simulink library "tpm"  (R2021b)
settings: Solver=VariableStepAuto  StartTime=0.0  StopTime=10.0  RelTol=1e-3
undefined symbols (not defined in the file or in its folder): ENUM_AN_LF, ENUM_AN_LR, ENUM_AN_RF, ENUM_AN_RR, ENUM_POWERSTA_OFF, ENUM_POWERSTA_OFFA, ENUM_POWERSTA_OFFC, ENUM_POWERSTA_ON, ENUM_POWERSTA_READY, ENUM_POWERSTA_STANDBY, ENUM_PWRSTASW_OFF, ENUM_PWRSTASW_OFFA, ENUM_PWRSTASW_OFFCHVCHRG, ENUM_PWRSTASW_STANDBY, FALSE, KTPM_Delay_raw8, KTPM_WhlRotDir_enum_ovrdflg, KTPM_WhlRotDir_enum_ovrdval, TRUE, ZERO_FLOAT, ZERO_INT
libraries: simulink x58, hcu_lib x25, $bdroot x18
(part 4 of 8)

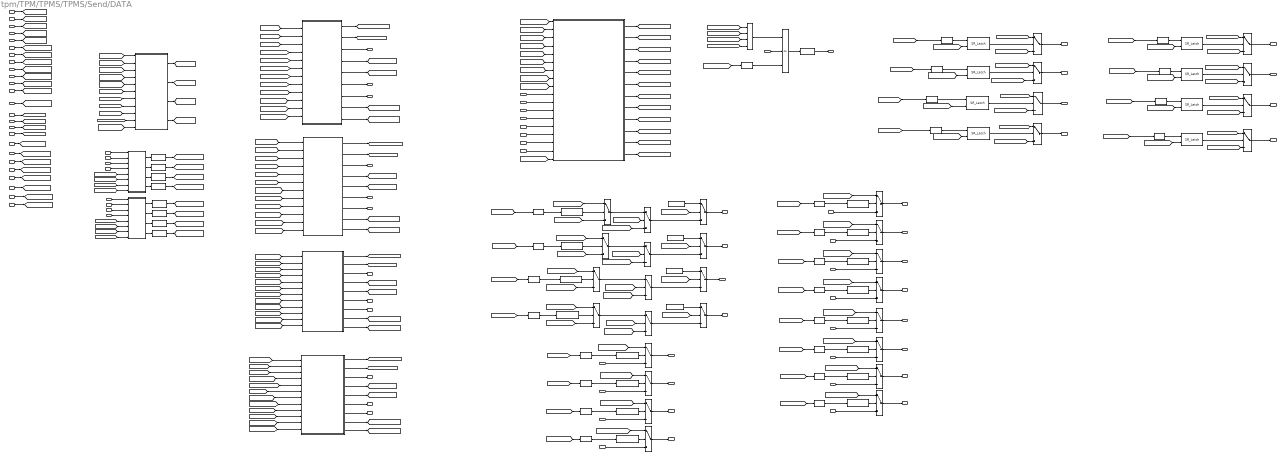
== system tpm/TPM/TPMS/TPMS/Send/DATA ==
  VPMM_PowerSta_enum : Inport
  VTPM_S1ID_raw32 : Inport  Port=2
  VTPM_S2ID_raw32 : Inport  Port=3
  VTPM_S3ID_raw32 : Inport  Port=4
  VTPM_S4ID_raw32 : Inport  Port=5
  VINP_IDin_raw32 : Inport  Port=6
  VINP_DATAin_flg : Inport  Port=7
  VTPM_Done_flg : Inport  Port=8
  VINP_Pin_raw8 : Inport  Port=9
  VINP_Tin_raw8 : Inport  Port=10
  VINP_BatteryLow_flg : Inport  Port=11
  VTPM_S1L_enum : Inport  Port=12
  VTPM_S2L_enum : Inport  Port=13
  VTPM_S3L_enum : Inport  Port=14
  VTPM_S4L_enum : Inport  Port=15
  VINP_FAT_flg : Inport  Port=16
  VINP_VehSpeed_kph : Inport  Port=17
  P1alarm : Inport  Port=18
  P1LowPindi : Inport  Port=19
  P2alarm : Inport  Port=20
  P2LowPindi : Inport  Port=21
  P3alarm : Inport  Port=22
  P3LowPindi : Inport  Port=23
  P4alarm : Inport  Port=24
  P4LowPindi : Inport  Port=25
  VTPM_IDLOCK_flg : Inport  Port=26
  VINP_TPMSResButt_flg : Inport  Port=27
  VINP_FlashLFSensorFail_flg : Inport  Port=28
  VINP_FlashRFSensorFail_flg : Inport  Port=29
  VINP_FlashLRSensorFail_flg : Inport  Port=30
  VINP_FlashRRSensorFail_flg : Inport  Port=31
  VINP_FlashLFWheelPress_raw8 : Inport  Port=32
  VINP_FlashRFWheelPress_raw8 : Inport  Port=33
  VINP_FlashLRFWheelPress_raw8 : Inport  Port=34
  VINP_FlashRRWheelPress_raw8 : Inport  Port=35
  VINP_FlashLFWheelTemp_C : Inport  Port=36
  VINP_FlashRFWheelTemp_C : Inport  Port=37
  VINP_FlashLRWheelTemp_C : Inport  Port=38
  VINP_FlashRRWheelTemp_C : Inport  Port=39
  VINP_FlashLFWheelPSW_raw8 : Inport  Port=40
  VINP_FlashRFWheelPSW_raw8 : Inport  Port=41
  VINP_FlashLRWheelPSW_raw8 : Inport  Port=42
  VINP_FlashRRWheelPSW_raw8 : Inport  Port=43
  VINP_FlashLFPindi_enum : Inport  Port=44
  VINP_FlashRFPindi_enum : Inport  Port=45
  VINP_FlashLRPindi_enum : Inport  Port=46
  VINP_FlashRRPindi_enum : Inport  Port=47
  VINP_FlashLFP20_raw8 : Inport  Port=48
  VINP_FlashRFP20_raw8 : Inport  Port=49
  VINP_FlashLRP20_raw8 : Inport  Port=50
  VINP_FlashRRP20_raw8 : Inport  Port=51
  VTPM_unlearnSfali_flg : Inport  Port=52
  VINP_TPMSCaliButt_flg : Inport  Port=53
  VINP_Prepresstemptrust_flg : Inport  Port=54
  Chart : Stateflow chart  TreatAsAtomicUnit=on
      settings: PortSchema="{\"entries\":[{\"content\":{\"sides\":[{\"content\":{\"connectorIds\":[\"In1\",\"In2\",\"In3\",\"In4\",\"In5\",\"In6\",\"In7\",\"In8\",\"In9\",\"In10\",\"In11\",\"In12\",\"In13\",\"In14\",\"In15\",\"In16\",\"In17\",\"In18\"]},\"type\":\"ConnectorPlacement.EquallySpacedRectSide\",\"uuid\":\"c40bc95c-7acd-49a7-a37f-73ef0237d825\"},{\"content\":{\"connectorIds\":[\"Out1\",\"Out2\",\"Out4\",\"Out3\",\"Out5\",\"Out6\",\"Out7\",\"Out8\",\"Out9\",\"Out10\",\"Out11\",\"Out12\"],\"side\":\"RIGHT\"},\"type\":\"ConnectorPlacement.EquallySpacedRectSide\",\"uuid\":\"6a475380-135f-4803-89fe-753926ba4981\"},{\"content\":{\"connectorIds\":[],\"side\":\"TOP\"},\"type\":\"ConnectorPlacement.EquallySpacedRectSide\",\"uuid\":\"32aff296-3980-42ee-80be-46132fdc59e9\"}]},\"type\":\"ConnectorPlacement.EquallySpacedConnector\",\"uuid\":\"d7f65336-a750-4257-81a4-fde8f4e67659\"}],\"packageUris\":[\"http://schema.mathworks.com/mf0/Connector/R2020b\"],\"version\":\"1.0\"}"
  Constant{1..4} (4 alike) : Constant  Value=TRUE
  Data Type Conversion{4..11,32} (9 alike) : DataTypeConversion  OutDataTypeStr=uint8
  Detect Increase{1..25} (25 alike) : simulink/Logic and Bit Operations/Detect Increase  vinit=0.0  OutDataTypeStr=boolean
  LFSW : Stateflow chart  TreatAsAtomicUnit=on
  LPindSwitch : MATLAB Function  TreatAsAtomicUnit=on
  LRSW : Stateflow chart  TreatAsAtomicUnit=on
      settings: PortSchema="{\"entries\":[{\"content\":{\"sides\":[{\"content\":{\"connectorIds\":[\"In1\",\"In2\",\"In3\",\"In4\",\"In5\",\"In6\",\"In8\",\"In7\",\"In9\",\"In10\",\"In11\",\"In12\"]},\"type\":\"ConnectorPlacement.EquallySpacedRectSide\",\"uuid\":\"46ef0c5c-df75-4382-9dd7-41a48e947ba5\"},{\"content\":{\"connectorIds\":[\"Out1\",\"Out2\",\"Out3\",\"Out4\",\"Out5\",\"Out6\",\"Out7\",\"Out8\",\"Out9\"],\"side\":\"RIGHT\"},\"type\":\"ConnectorPlacement.EquallySpacedRectSide\",\"uuid\":\"b740a0a9-c0c3-4741-b0bb-461f50318db6\"},{\"content\":{\"connectorIds\":[],\"side\":\"TOP\"},\"type\":\"ConnectorPlacement.EquallySpacedRectSide\",\"uuid\":\"ad8490db-8659-4e68-a885-1504b96317d8\"}]},\"type\":\"ConnectorPlacement.EquallySpacedConnector\",\"uuid\":\"0b7e90cb-07df-4d51-93f4-cbf71996ee01\"}],\"packageUris\":[\"http://schema.mathworks.com/mf0/Connector/R2020b\"],\"version\":\"1.0\"}"
  Latch{4..19} (16 alike) : hcu_lib/Basic_Blocks/Latch
  LocationSW : Subsystem
  Logical Operator1 : Logic  Inputs=4  AllPortsSameDT=off  OutDataTypeStr=boolean
  Logical Operator2 : Logic  Operator=OR  Inputs=3  AllPortsSameDT=off  OutDataTypeStr=boolean
  PalarmSwitch : MATLAB Function  TreatAsAtomicUnit=on
  RFSW : Stateflow chart  TreatAsAtomicUnit=on
  RRSW : Stateflow chart  TreatAsAtomicUnit=on
  SR_Latch{,1..7} (8 alike) : hcu_lib/Basic_Blocks/SR_Latch
  Switch{,1..31} (32 alike) : Switch  Criteria=u2 ~= 0
  VTPM_LFWheelPress_raw8 : Outport
  VTPM_LFWheelTemp_C : Outport  Port=2
  VTPM_LFBatWarn_flg : Outport  Port=3
  VTPM_RFWheelPress_raw8 : Outport  Port=4
  VTPM_RFWheelTemp_C : Outport  Port=5
  VTPM_RFBatWarn_flg : Outport  Port=6
  VTPM_LRWheelPress_raw8 : Outport  Port=7
  VTPM_LRWheelTemp_C : Outport  Port=8
  VTPM_LRBatWarn_flg : Outport  Port=9
  VTPM_RRWheelPress_raw8 : Outport  Port=10
  VTPM_RRWheelTemp_C : Outport  Port=11
  VTPM_RRBatWarn_flg : Outport  Port=12
  VTPM_LFWheelDebug_flg : Outport  Port=13
  VTPM_RFWheelDebug_flg : Outport  Port=14
  VTPM_LRWheelDebug_flg : Outport  Port=15
  VTPM_RRWheelDebug_flg : Outport  Port=16
  VTPM_LFSensorMode_flg : Outport  Port=17
  VTPM_RFSensorMode_flg : Outport  Port=18
  VTPM_LRSensorMode_flg : Outport  Port=19
  VTPM_RRSensorMode_flg : Outport  Port=20
  VTPM_LFSensorFail_flg : Outport  Port=21
  VTPM_RFSensorFail_flg : Outport  Port=22
  VTPM_LRSensorFail_flg : Outport  Port=23
  VTPM_RRSensorFail_flg : Outport  Port=24
  VTPM_LFP20_raw8 : Outport  Port=25
  VTPM_RFP20_raw8 : Outport  Port=26
  VTPM_LRP20_raw8 : Outport  Port=27
  VTPM_RRP20_raw8 : Outport  Port=28
  VTPM_LFWheelPSW_raw8 : Outport  Port=29
  VTPM_LFPindi_enum : Outport  Port=30
  VTPM_RFWheelPSW_raw8 : Outport  Port=31
  VTPM_RFPind_enum : Outport  Port=32
  VTPM_LRWheelPSW_raw8 : Outport  Port=33
  VTPM_LRPindi_enum : Outport  Port=34
  VTPM_RRWheelPSW_raw8 : Outport  Port=35
  VTPM_RRPindi_enum : Outport  Port=36
  VTPM_Prepresstempvalid_enum : Outport  Port=37
  wires:
  VINP_Pin_raw8/1 -> [VINP_Pin_raw8]
  VINP_Tin_raw8/1 -> [VINP_Tin_raw8]
  VINP_BatteryLow_flg/1 -> [VINP_BatteryLow_flg]
  LocationSW/1(VTPM_LFSW_flg) -> [VTPM_LFSW_flg]
  LocationSW/2(VTPM_RFSW_flg) -> [VTPM_RFSW_flg]
  LocationSW/3(VTPM_LRSW_flg) -> [VTPM_LRSW_flg]
  LocationSW/4(VTPM_RRSW_flg) -> [VTPM_RRSW_flg]
  VPMM_PowerSta_enum/1 -> [VPMM_PowerSta_enum]
  VINP_DATAin_flg/1 -> [VINP_DATAin_flg]
  VINP_FAT_flg/1 -> [VINP_FAT_flg]
  VINP_VehSpeed_kph/1 -> [VINP_VehSpeed_kph]
  [VINP_FAT_flg] -> LFSW/6(VINP_FAT_flg)
  [VPMM_PowerSta_enum] -> LFSW/5(VPMM_PowerSta_enum)
  [VINP_VehSpeed_kph] -> LFSW/9(VINP_VehSpeed_kph)
  [VTPM_Done_flg] -> LFSW/10(VTPM_Done_flg)
  [VINP_Pin_raw8] -> LFSW/2(VINP_Pin_raw8)
  [VINP_Tin_raw8] -> LFSW/3(VTPM_Tin_c)
  [VTPM_LFSW_flg] -> LFSW/1(VTPM_LFSW_flg)
  [VTPM_LFLowPind_raw] -> LFSW/8(VTPM_S1LowPindi_enum)
  [VINP_BatteryLow_flg] -> LFSW/4(VINP_BatteryLow_flg)
  [VTPM_LFPalarm_raw16] -> LFSW/7(VTPM_LFPalarm_raw16)
  [VTPM_S3L_enum] -> LPindSwitch/7(S3L)
  P4alarm/1 -> PalarmSwitch/4(P4)
  LPindSwitch/2(RFP) -> Data Type Conversion9/1
  [VTPM_S2L_enum] -> PalarmSwitch/6(S2L)
  [VTPM_S4L_enum] -> PalarmSwitch/8(S4L)
  PalarmSwitch/3(LRP) -> Data Type Conversion6/1
  P3LowPindi/1 -> LPindSwitch/3(P3)
  P4LowPindi/1 -> LPindSwitch/4(P4)
  [VTPM_S1L_enum] -> LPindSwitch/5(S1L)
  LPindSwitch/1(LFP) -> Data Type Conversion8/1
  LPindSwitch/4(RRP) -> Data Type Conversion11/1
  [VTPM_S2L_enum] -> LPindSwitch/6(S2L)
  P1LowPindi/1 -> LPindSwitch/1(P1)
  [VTPM_S4L_enum] -> LPindSwitch/8(S4L)
  P1alarm/1 -> PalarmSwitch/1(P1)
  [VTPM_S1L_enum] -> PalarmSwitch/5(S1L)
  PalarmSwitch/1(LFP) -> Data Type Conversion4/1
  [VTPM_S3L_enum] -> PalarmSwitch/7(S3L)
  PalarmSwitch/4(RRP) -> Data Type Conversion7/1
  PalarmSwitch/2(RFP) -> Data Type Conversion5/1
  LPindSwitch/3(LRP) -> Data Type Conversion10/1
  P2alarm/1 -> PalarmSwitch/2(P2)
  P2LowPindi/1 -> LPindSwitch/2(P2)
  P3alarm/1 -> PalarmSwitch/3(P3)
  Data Type Conversion4/1 -> [VTPM_LFPalarm_raw16]
  Data Type Conversion5/1 -> [VTPM_RFPalarm_raw16]
  Data Type Conversion6/1 -> [VTPM_LRPalarm_raw16]
  Data Type Conversion7/1 -> [VTPM_RRPalarm_raw16]
  Data Type Conversion8/1 -> [VTPM_LFLowPind_raw]
  Data Type Conversion9/1 -> [VTPM_RFLowPind_raw]
  Data Type Conversion10/1 -> [VTPM_LRLowPind_raw]
  Data Type Conversion11/1 -> [VTPM_RRLowPind_raw]
  VTPM_S1L_enum/1 -> [VTPM_S1L_enum]
  VTPM_S2L_enum/1 -> [VTPM_S2L_enum]
  VTPM_S3L_enum/1 -> [VTPM_S3L_enum]
  VTPM_S4L_enum/1 -> [VTPM_S4L_enum]
  LFSW/3(VTPM_LFBatWarn_flg) -> VTPM_LFBatWarn_flg/1
  LFSW/6(VTPM_LFWheelDebug_flg) -> VTPM_LFWheelDebug_flg/1
  LFSW/7(VTPM_LFSensorMode_flg) -> VTPM_LFSensorMode_flg/1
  [VINP_DATAin_flg] -> LocationSW/10(VINP_DATAin_flg)
  [VTPM_S1L_enum] -> LocationSW/6(VTPM_S1L_enum)
  [VTPM_S2L_enum] -> LocationSW/7(VTPM_S2L_enum)
  [VTPM_S3L_enum] -> LocationSW/8(VTPM_S3L_enum)
  [VTPM_S4L_enum] -> LocationSW/9(VTPM_S4L_enum)
  VTPM_Done_flg/1 -> [VTPM_Done_flg]
  [VTPM_IDLOCK_flg] -> LocationSW/11(VTPM_IDLOCK_flg)
  VTPM_S1ID_raw32/1 -> [VTPM_S1ID_raw32]
  VTPM_S2ID_raw32/1 -> [VTPM_S2ID_raw32]
  VTPM_S3ID_raw32/1 -> [VTPM_S3ID_raw32]
  VTPM_S4ID_raw32/1 -> [VTPM_S4ID_raw32]
  VINP_IDin_raw32/1 -> [VINP_IDin_raw32]
  [VTPM_S4ID_raw32] -> LocationSW/4(VTPM_S4ID_raw32)
  [VTPM_S3ID_raw32] -> LocationSW/3(VTPM_S3ID_raw32)
  [VINP_IDin_raw32] -> LocationSW/5(VINP_IDin_raw32)
  [VTPM_S2ID_raw32] -> LocationSW/2(VTPM_S2ID_raw32)
  [VTPM_S1ID_raw32] -> LocationSW/1(VTPM_S1ID_raw32)
  [VTPM_S3ID_raw32] -> Chart/4(VTPM_S3ID_raw32)
  [VTPM_S2ID_raw32] -> Chart/3(VTPM_S2ID_raw32)
  [VTPM_S4ID_raw32] -> Chart/5(VTPM_S4ID_raw32)
  [VTPM_S1ID_raw32] -> Chart/2(VTPM_S1ID_raw32)
  [VINP_IDin_raw32] -> Chart/6(VINP_IDin_raw32)
  [VINP_Pin_raw8] -> Chart/8(VINP_Pin_raw8)
  [VINP_DATAin_flg] -> Chart/1(VINP_DATAin_flg)
  VTPM_IDLOCK_flg/1 -> [VTPM_IDLOCK_flg]
  [VTPM_IDLOCK_flg] -> Chart/7(VTPM_IDLOCK_flg)
  [VINP_Tin_raw8] -> Chart/9(VINP_Tin_raw8)
  Chart/1(VTPM_PreS1Pressure_raw) -> [VTPM_PreS1Pressure_raw]
  Chart/2(VTPM_PreS2Pressure_raw) -> [VTPM_PreS2Pressure_raw]
  Chart/5(VTPM_PreS1Temp_raw) -> [VTPM_PreS1Temp_raw]
  Chart/6(VTPM_PreS2Temp_raw) -> [VTPM_PreS2Temp_raw]
  Chart/7(VTPM_PreS3Temp_raw) -> [VTPM_PreS3Temp_raw]
  Chart/8(VTPM_PreS4Temp_raw) -> [VTPM_PreS4Temp_raw]
  Chart/4(VTPM_PreS3Pressure_raw) -> [VTPM_PreS3Pressure_raw]
  Chart/3(VTPM_PreS4Pressure_raw) -> [VTPM_PreS4Pressure_raw]
  LFSW/4(VTPM_LFSensorFail_flg) -> [VTPM_LFSensorFail_flg]
  LFSW/5(VTPM_LFP20_raw8) -> [VTPM_LFP20_raw8]
  LFSW/8(VTPM_LFWheelPSW_raw8) -> [VTPM_LFWheelPSW_raw8]
  LFSW/9(VTPM_LFPindi_enum) -> [VTPM_LFPindi_enum]
  VINP_FlashLFSensorFail_flg/1 -> [VINP_FlashLFSensorFail_flg]
  VINP_FlashRFSensorFail_flg/1 -> [VINP_FlashRFSensorFail_flg]
  VINP_FlashLRSensorFail_flg/1 -> [VINP_FlashLRSensorFail_flg]
  VINP_FlashRRSensorFail_flg/1 -> [VINP_FlashRRSensorFail_flg]
  VINP_FlashLFWheelPress_raw8/1 -> Chart/10(VINP_FlashLFWheelPress_raw8)
  VINP_FlashRFWheelPress_raw8/1 -> Chart/11(VINP_FlashRFWheelPress_raw8)
  VINP_FlashLRFWheelPress_raw8/1 -> Chart/12(VINP_FlashLRWheelPress_raw8)
  VINP_FlashRRWheelPress_raw8/1 -> Chart/13(VINP_FlashRRWheelPress_raw8)
  VINP_FlashLFWheelTemp_C/1 -> Chart/14(VINP_FlashLFWheelTemp_C)
  VINP_FlashRFWheelTemp_C/1 -> Chart/15(VINP_FlashRFWheelTemp_C)
  VINP_FlashLRWheelTemp_C/1 -> Chart/16(VINP_FlashLRWheelTemp_C)
  VINP_FlashRRWheelTemp_C/1 -> Chart/17(VINP_FlashRRWheelTemp_C)
  Switch15/1 -> VTPM_RRPindi_enum/1
  Switch10/1 -> VTPM_LRWheelPSW_raw8/1
  Switch14/1 -> VTPM_LRPindi_enum/1
  Switch11/1 -> VTPM_RRWheelPSW_raw8/1
  Switch4/1 -> VTPM_LFP20_raw8/1
  Switch7/1 -> VTPM_RRP20_raw8/1
  Switch5/1 -> VTPM_RFP20_raw8/1
  Switch8/1 -> VTPM_LFWheelPSW_raw8/1
  Switch13/1 -> VTPM_RFPind_enum/1
  Switch6/1 -> VTPM_LRP20_raw8/1
  Switch9/1 -> VTPM_RFWheelPSW_raw8/1
  Switch12/1 -> VTPM_LFPindi_enum/1
  VINP_FlashRRP20_raw8/1 -> Switch7/3
  VINP_FlashLRPindi_enum/1 -> Switch14/3
  VINP_FlashRRWheelPSW_raw8/1 -> Switch11/3
  VINP_FlashLFWheelPSW_raw8/1 -> Switch8/3
  VINP_FlashRFP20_raw8/1 -> Switch5/3
  VINP_FlashLFP20_raw8/1 -> Switch4/3
  VINP_FlashRRPindi_enum/1 -> Switch15/3
  VINP_FlashRFPindi_enum/1 -> Switch13/3
  VINP_FlashLFPindi_enum/1 -> Switch12/3
  Switch3/1 -> Switch19/1
  Detect Increase4/1 -> Latch4/1
  VINP_FlashRFWheelPSW_raw8/1 -> Switch9/3
  Detect Increase19/1 -> Latch19/1
  [VTPM_LRSW_flg] -> Detect Increase10/1
  [VTPM_RRSW_flg] -> Detect Increase19/1
  Latch13/1 -> Switch9/2
  [VTPM_RRSensorFail_flg] -> Switch19/3
  Latch17/1 -> Switch13/2
  [VTPM_LRPindi_enum] -> Switch14/1
  Latch16/1 -> Switch12/2
  [VTPM_LFP20_raw8] -> Switch4/1
  [VINP_FlashRRSensorFail_flg] -> Switch3/3
  Detect Increase13/1 -> Latch13/1
  [VINP_FlashRRSensorFail_flg] -> Switch19/2
  [VINP_FlashLRSensorFail_flg] -> Switch2/3
  [VTPM_RFPind_enum] -> Switch13/1
  [VTPM_LFSW_flg] -> Detect Increase16/1
  [VTPM_RFSW_flg] -> Detect Increase17/1
  Switch2/1 -> Switch18/1
  [VINP_FlashLRSensorFail_flg] -> Switch18/2
  [VTPM_RFSensorFail_flg] -> Switch1/1
  [VTPM_LRSensorFail_flg] -> Switch18/3
  [VINP_FlashRFSensorFail_flg] -> Switch17/2
  [VINP_FlashRFSensorFail_flg] -> Switch1/3
  [VTPM_RRSensorFail_flg] -> Switch3/1
  Detect Increase8/1 -> Latch8/1
  [VINP_FlashLFSensorFail_flg] -> Switch/3
  Latch9/1 -> Switch5/2
  Detect Increase18/1 -> Latch18/1
  [VTPM_RFSW_flg] -> Detect Increase9/1
  [VTPM_RFSW_flg] -> Detect Increase5/1
  Switch/1 -> Switch16/1
  [VTPM_LFSensorFail_flg] -> Switch16/3
  [VTPM_RFSW_flg] -> Detect Increase13/1
  [VTPM_RRWheelPSW_raw8] -> Switch11/1
  Latch18/1 -> Switch14/2
  Detect Increase14/1 -> Latch14/1
  [VTPM_LRSW_flg] -> Detect Increase18/1
  Detect Increase15/1 -> Latch15/1
  [VTPM_RRSW_flg] -> Detect Increase15/1
  VINP_FlashLRP20_raw8/1 -> Switch6/3
  [VTPM_RFP20_raw8] -> Switch5/1
  [VTPM_RRSW_flg] -> Detect Increase11/1
  Detect Increase17/1 -> Latch17/1
  Detect Increase16/1 -> Latch16/1
  Latch19/1 -> Switch15/2
  Detect Increase10/1 -> Latch10/1
  Latch12/1 -> Switch8/2
  Latch11/1 -> Switch7/2
  Detect Increase9/1 -> Latch9/1
  Latch7/1 -> Switch3/2
  [VTPM_LRSW_flg] -> Detect Increase6/1
  [VTPM_RRP20_raw8] -> Switch7/1
  [VTPM_LFSW_flg] -> Detect Increase8/1
  [VINP_FlashLFSensorFail_flg] -> Switch16/2
  [VTPM_RFWheelPSW_raw8] -> Switch9/1
  Detect Increase11/1 -> Latch11/1
  Detect Increase5/1 -> Latch5/1
  [VTPM_RFSensorFail_flg] -> Switch17/3
  Latch15/1 -> Switch11/2
  Latch6/1 -> Switch2/2
  Latch4/1 -> Switch/2
  Latch14/1 -> Switch10/2
  [VTPM_LRP20_raw8] -> Switch6/1
  Detect Increase6/1 -> Latch6/1
  Switch1/1 -> Switch17/1
  [VTPM_LFPindi_enum] -> Switch12/1
  [VTPM_LRSW_flg] -> Detect Increase14/1
  Latch10/1 -> Switch6/2
  [VTPM_RRPindi_enum] -> Switch15/1
  VINP_FlashLRWheelPSW_raw8/1 -> Switch10/3
  Latch8/1 -> Switch4/2
  [VTPM_LFWheelPSW_raw8] -> Switch8/1
  [VTPM_LFSW_flg] -> Detect Increase4/1
  [VTPM_LFSensorFail_flg] -> Switch/1
  Detect Increase12/1 -> Latch12/1
  [VTPM_LRSensorFail_flg] -> Switch2/1
  [VTPM_LFSW_flg] -> Detect Increase12/1
  Detect Increase7/1 -> Latch7/1
  Latch5/1 -> Switch1/2
  [VTPM_RRSW_flg] -> Detect Increase7/1
  [VTPM_LRWheelPSW_raw8] -> Switch10/1
  VTPM_unlearnSfali_flg/1 -> [VTPM_unlearnSfali_flg]
  Switch16/1 -> Switch20/3
  Switch17/1 -> Switch21/3
  Switch18/1 -> Switch22/3
  Switch19/1 -> Switch23/3
  [VTPM_unlearnSfali_flg] -> Switch20/2
  [VTPM_unlearnSfali_flg] -> Switch21/2
  [VTPM_unlearnSfali_flg] -> Switch22/2
  [VTPM_unlearnSfali_flg] -> Switch23/2
  Constant4/1 -> Switch23/1
  Constant1/1 -> Switch22/1
  Constant2/1 -> Switch21/1
  Constant3/1 -> Switch20/1
  Switch20/1 -> VTPM_LFSensorFail_flg/1
  Switch21/1 -> VTPM_RFSensorFail_flg/1
  Switch22/1 -> VTPM_LRSensorFail_flg/1
  Switch23/1 -> VTPM_RRSensorFail_flg/1
  Data Type Conversion32/1 -> VTPM_Prepresstempvalid_enum/1
  VINP_TPMSCaliButt_flg/1 -> [VINP_TPMSCaliButt_flg]
  VINP_TPMSResButt_flg/1 -> [VINP_TPMSResButt_flg]
  [VINP_TPMSCaliButt_flg] -> LFSW/11(VINP_TPMSCaliButt_flg)
  [VINP_TPMSResButt_flg] -> LFSW/12(VINP_TPMSResButt_flg)
  [VTPM_RFPalarm_raw16] -> RFSW/7(VTPM_P2alarm_raw16)
  [VTPM_RFLowPind_raw] -> RFSW/8(VTPM_S2LowPindi_enum)
  [VINP_VehSpeed_kph] -> RFSW/9(VINP_VehSpeed_kph)
  [VTPM_Done_flg] -> RFSW/10(VTPM_Done_flg)
  [VTPM_RFSW_flg] -> RFSW/1(VTPM_RFSW_flg)
  [VINP_Pin_raw8] -> RFSW/2(VINP_Pin_raw8)
  [VINP_Tin_raw8] -> RFSW/3(VTPM_Tin_c)
  [VINP_BatteryLow_flg] -> RFSW/4(VINP_BatteryLow_flg)
  [VPMM_PowerSta_enum] -> RFSW/5(VPMM_PowerSta_enum)
  [VINP_FAT_flg] -> RFSW/6(VINP_FAT_flg)
  [VTPM_LRSW_flg] -> LRSW/1(VTPM_LRSW_flg)
  [VINP_Pin_raw8] -> LRSW/2(VINP_Pin_raw8)
  [VINP_Tin_raw8] -> LRSW/3(VTPM_Tin_c)
  [VINP_BatteryLow_flg] -> LRSW/4(VINP_BatteryLow_flg)
  [VPMM_PowerSta_enum] -> LRSW/5(VPMM_PowerSta_enum)
  [VINP_FAT_flg] -> LRSW/6(VINP_FAT_flg)
  [VINP_VehSpeed_kph] -> LRSW/9(VINP_VehSpeed_kph)
  [VTPM_Done_flg] -> LRSW/10(VTPM_Done_flg)
  [VTPM_LRPalarm_raw16] -> LRSW/8(VTPM_P3alarm_raw16)
  [VTPM_LRLowPind_raw] -> LRSW/7(VTPM_S3LowPindi_enum)
  [VPMM_PowerSta_enum] -> RRSW/5(VPMM_PowerSta_enum)
  [VTPM_RRLowPind_raw] -> RRSW/8(VTPM_S4LowPindi_enum)
  [VTPM_Done_flg] -> RRSW/10(VTPM_Done_flg)
  [VINP_BatteryLow_flg] -> RRSW/4(VINP_BatteryLow_flg)
  [VINP_VehSpeed_kph] -> RRSW/9(VINP_VehSpeed_kph)
  [VTPM_RRPalarm_raw16] -> RRSW/7(VTPM_P4alarm_raw16)
  [VTPM_RRSW_flg] -> RRSW/1(VTPM_RRSW_flg)
  [VINP_Pin_raw8] -> RRSW/2(VINP_Pin_raw8)
  [VINP_Tin_raw8] -> RRSW/3(VTPM_Tin_c)
  [VINP_FAT_flg] -> RRSW/6(VINP_FAT_flg)
  RFSW/9(VTPM_RFPind_enum) -> [VTPM_RFPind_enum]
  RFSW/3(VTPM_RFBatWarn_flg) -> VTPM_RFBatWarn_flg/1
  RFSW/4(VTPM_RFSensorFail_flg) -> [VTPM_RFSensorFail_flg]
  RFSW/5(VTPM_RFP20_raw8) -> [VTPM_RFP20_raw8]
  RFSW/6(VTPM_RFWheelDebug_flg) -> VTPM_RFWheelDebug_flg/1
  RFSW/7(VTPM_RFSensorMode_flg) -> VTPM_RFSensorMode_flg/1
  RFSW/8(VTPM_RFWheelPSW_raw8) -> [VTPM_RFWheelPSW_raw8]
  LRSW/3(VTPM_LRBatWarn_flg) -> VTPM_LRBatWarn_flg/1
  LRSW/4(VTPM_LRSensorFail_flg) -> [VTPM_LRSensorFail_flg]
  LRSW/5(VTPM_LRP20_raw8) -> [VTPM_LRP20_raw8]
  LRSW/6(VTPM_LRWheelDebug_flg) -> VTPM_LRWheelDebug_flg/1
  LRSW/7(VTPM_LRSensorMode_flg) -> VTPM_LRSensorMode_flg/1
  LRSW/8(VTPM_LRWheelPSW_raw8) -> [VTPM_LRWheelPSW_raw8]
  LRSW/9(VTPM_LRPindi_enum) -> [VTPM_LRPindi_enum]
  RRSW/3(VTPM_RRBatWarn_flg) -> VTPM_RRBatWarn_flg/1
  RRSW/4(VTPM_RRSensorFail_flg) -> [VTPM_RRSensorFail_flg]
  RRSW/5(VTPM_RRP20_raw8) -> [VTPM_RRP20_raw8]
  RRSW/6(VTPM_RRWheelDebug_flg) -> VTPM_RRWheelDebug_flg/1
  RRSW/7(VTPM_RRSensorMode_flg) -> VTPM_RRSensorMode_flg/1
  RRSW/8(VTPM_RRWheelPSW_raw8) -> [VTPM_RRWheelPSW_raw8]
  RRSW/9(VTPM_RRPindi_enum) -> [VTPM_RRPindi_enum]
  [VINP_TPMSCaliButt_flg] -> RFSW/11(VINP_TPMSCaliButt_flg)
  [VINP_TPMSResButt_flg] -> RFSW/12(VINP_TPMSResButt_flg)
  [VINP_TPMSCaliButt_flg] -> LRSW/11(VINP_TPMSCaliButt_flg)
  [VINP_TPMSResButt_flg] -> LRSW/12(VINP_TPMSResButt_flg)
  [VINP_TPMSCaliButt_flg] -> RRSW/11(VINP_TPMSCaliButt_flg)
  [VINP_TPMSResButt_flg] -> RRSW/12(VINP_TPMSResButt_flg)
  [VINP_TPMSResButt_flg] -> Chart/18(VINP_TPMSResButt_flg)
  LFSW/1(VTPM_LFWheelPress_raw8) -> [VTPM_LFWheelPress_raw8]
  LFSW/2(VTPM_LFWheelTemp_C) -> [VTPM_LFWheelTemp_C]
  RFSW/2(VTPM_RFWheelTemp_C) -> [VTPM_RFWheelTemp_C]
  RFSW/1(VTPM_RFWheelPress_raw8) -> [VTPM_RFWheelPress_raw8]
  LRSW/1(VTPM_LRWheelPress_raw8) -> [VTPM_LRWheelPress_raw8]
  LRSW/2(VTPM_LRWheelTemp_C) -> [VTPM_LRWheelTemp_C]
  RRSW/1(VTPM_RRWheelPress_raw8) -> [VTPM_RRWheelPress_raw8]
  RRSW/2(VTPM_RRWheelTemp_C) -> [VTPM_RRWheelTemp_C]
  [VTPM_LFSW_flg] -> Detect Increase21/1
  Detect Increase22/1 -> SR_Latch3/1
  [VTPM_RFSW_flg] -> Detect Increase22/1
  SR_Latch2/1 -> Switch28/2
  [VTPM_PreS1Temp_raw] -> Switch28/3
  [VTPM_PreS1Pressure_raw] -> Switch24/3
  SR_Latch1/1 -> Switch25/2
  Detect Increase21/1 -> SR_Latch2/1
  [VTPM_RFSW_flg] -> Detect Increase2/1
  [VTPM_LFSW_flg] -> Detect Increase1/1
  [VTPM_RFWheelTemp_C] -> Switch29/1
  [VTPM_PreS2Temp_raw] -> Switch29/3
  Detect Increase2/1 -> SR_Latch1/1
  [VTPM_LFWheelPress_raw8] -> Switch24/1
  [VTPM_LFWheelTemp_C] -> Switch28/1
  [VTPM_RFWheelPress_raw8] -> Switch25/1
  [VTPM_PreS2Pressure_raw] -> Switch25/3
  [VTPM_LRWheelPress_raw8] -> Switch26/1
  [VTPM_LRSW_flg] -> Detect Increase3/1
  [VTPM_RRWheelTemp_C] -> Switch31/1
  [VTPM_LRSW_flg] -> Detect Increase23/1
  [VTPM_PreS4Temp_raw] -> Switch31/3
  [VTPM_RRSW_flg] -> Detect Increase24/1
  SR_Latch6/1 -> Switch30/2
  [VTPM_RRWheelPress_raw8] -> Switch27/1
  [VTPM_LRWheelTemp_C] -> Switch30/1
  [VTPM_PreS3Temp_raw] -> Switch30/3
  [VTPM_PreS3Pressure_raw] -> Switch26/3
  [VTPM_PreS4Pressure_raw] -> Switch27/3
  [VTPM_RRSW_flg] -> Detect Increase20/1
  Switch24/1 -> VTPM_LFWheelPress_raw8/1
  Switch28/1 -> VTPM_LFWheelTemp_C/1
  Switch25/1 -> VTPM_RFWheelPress_raw8/1
  Switch29/1 -> VTPM_RFWheelTemp_C/1
  Switch26/1 -> VTPM_LRWheelPress_raw8/1
  Switch30/1 -> VTPM_LRWheelTemp_C/1
  Switch27/1 -> VTPM_RRWheelPress_raw8/1
  Switch31/1 -> VTPM_RRWheelTemp_C/1
  Chart/12(VTPM_PreS4readdone_flg) -> [VTPM_PreS4readdone_flg]
  Chart/11(VTPM_PreS3readdone_flg) -> [VTPM_PreS3readdone_flg]
  Chart/10(VTPM_PreS2readdone_flg) -> [VTPM_PreS2readdone_flg]
  Chart/9(VTPM_PreS1readdone_flg) -> [VTPM_PreS1readdone_flg]
  [VTPM_PreS1readdone_flg] -> Logical Operator1/1
  [VTPM_PreS3readdone_flg] -> Logical Operator1/3
  [VTPM_PreS2readdone_flg] -> Logical Operator1/2
  [VTPM_PreS4readdone_flg] -> Logical Operator1/4
  Logical Operator1/1 -> Logical Operator2/1
  Logical Operator2/1 -> Data Type Conversion32/1
  VINP_Prepresstemptrust_flg/1 -> Logical Operator2/2
  [VINP_TPMSResButt_flg] -> SR_Latch/2
  Detect Increase1/1 -> SR_Latch/1
  SR_Latch/1 -> Switch24/2
  [VINP_TPMSResButt_flg] -> SR_Latch1/2
  [VINP_TPMSResButt_flg] -> SR_Latch2/2
  [VINP_TPMSResButt_flg] -> SR_Latch3/2
  SR_Latch3/1 -> Switch29/2
  [VINP_TPMSResButt_flg] -> SR_Latch4/2
  Detect Increase3/1 -> SR_Latch4/1
  SR_Latch4/1 -> Switch26/2
  [VINP_TPMSResButt_flg] -> SR_Latch5/2
  Detect Increase20/1 -> SR_Latch5/1
  SR_Latch5/1 -> Switch27/2
  [VINP_TPMSResButt_flg] -> SR_Latch6/2
  Detect Increase23/1 -> SR_Latch6/1
  [VINP_TPMSResButt_flg] -> SR_Latch7/2
  Detect Increase24/1 -> SR_Latch7/1
  SR_Latch7/1 -> Switch31/2
  [VINP_TPMSResButt_flg] -> Detect Increase25/1
  Detect Increase25/1 -> Logical Operator2/3

== system tpm/TPM/TPMS/TPMS/Send/ResetAllow&CalibrateAllow ==
  VTQD_GearActualPosn_enum : Inport
  VINP_VehSpeed_kph : Inport  Port=2
  VINP_TPMSResButt_flg : Inport  Port=3
  VINP_TPMSCaliButt_flg : Inport  Port=4
  VTPM_Done_flg : Inport  Port=5
  Chart : Stateflow chart  TreatAsAtomicUnit=on
      settings: PortSchema="{\"entries\":[{\"content\":{\"sides\":[{\"content\":{\"connectorIds\":[\"In1\",\"In2\",\"In3\",\"In4\",\"In5\"]},\"type\":\"ConnectorPlacement.EquallySpacedRectSide\",\"uuid\":\"5043c8d7-7d74-4216-81db-b94b6209e2f2\"},{\"content\":{\"connectorIds\":[\"Out2\",\"Out1\"],\"side\":\"RIGHT\"},\"type\":\"ConnectorPlacement.EquallySpacedRectSide\",\"uuid\":\"32f8b1e1-37fd-4ec2-8559-79f51e6b5aad\"},{\"content\":{\"connectorIds\":[],\"side\":\"TOP\"},\"type\":\"ConnectorPlacement.EquallySpacedRectSide\",\"uuid\":\"4b4c5b66-4800-4ce6-9315-053bf75e645c\"}]},\"type\":\"ConnectorPlacement.EquallySpacedConnector\",\"uuid\":\"baa92019-e8c5-41db-ba73-e08b6ede8e32\"}],\"packageUris\":[\"http://schema.mathworks.com/mf0/Connector/R2020b\"],\"version\":\"1.0\"}"
  VTPM_TPMSResButtAllow_flg : Outport
  VTPM_TPMSCaliButtAllow_flg : Outport  Port=2
  wires:
  VINP_TPMSCaliButt_flg/1 -> Chart/4(VINP_TPMSCaliButt_flg)
  VTPM_Done_flg/1 -> Chart/5(VTPM_Done_flg)
  Chart/1(VTPM_TPMSCaliButtAllow_flg) -> VTPM_TPMSCaliButtAllow_flg/1
  Chart/2(VTPM_TPMSResButtAllow_flg) -> VTPM_TPMSResButtAllow_flg/1
  VINP_TPMSResButt_flg/1 -> Chart/3(VINP_TPMSResButt_flg)
  VINP_VehSpeed_kph/1 -> Chart/2(VINP_VehSpeed_kph)
  VTQD_GearActualPosn_enum/1 -> Chart/1(VTQD_GearActualPosn_enum)

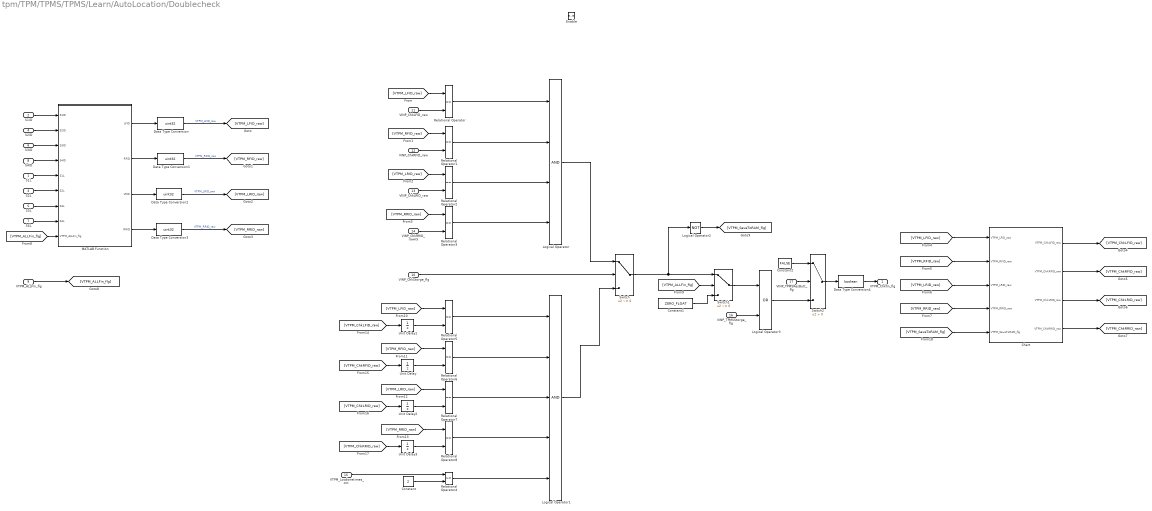
== system tpm/TPM/TPMS/TPMS/Learn/AutoLocation/Doublecheck ==
  S1L : Inport
  S1ID : Inport  Port=2
  S2L : Inport  Port=3
  S2ID : Inport  Port=4
  S3L : Inport  Port=5
  S3ID : Inport  Port=6
  S4L : Inport  Port=7
  S4ID : Inport  Port=8
  VTPM_ALLFin_flg : Inport  Port=9
  VINP_ChkStorge_flg : Inport  Port=10
  VINP_ChkLFID_raw : Inport  Port=11
  VINP_ChkRFID_raw : Inport  Port=12
  VINP_ChkLRID_raw : Inport  Port=13
  VINP_ChkRRID_rawn5 : Inport  Port=14
  VTPM_Locdonetimes_cnt : Inport  Port=15
  VINP_TPMSStorge_flg : Inport  Port=16
  VINP_TPMSResButt_flg : Inport  Port=17
  Enable : EnablePort
  Chart : Stateflow chart  TreatAsAtomicUnit=on
  Constant : Constant  Value=2
  Constant1 : Constant  Value=ZERO_FLOAT
  Constant2 : Constant  Value=FALSE
  Data Type Conversion{,1..3} (4 alike) : DataTypeConversion  OutDataTypeStr=uint32
  Data Type Conversion4 : DataTypeConversion  OutDataTypeStr=boolean
  Logical Operator : Logic  Inputs=4  AllPortsSameDT=off  OutDataTypeStr=boolean
  Logical Operator1 : Logic  Inputs=5  AllPortsSameDT=off  OutDataTypeStr=boolean
  Logical Operator2 : Logic  Operator=NOT  AllPortsSameDT=off  OutDataTypeStr=boolean
  Logical Operator3 : Logic  Operator=OR  AllPortsSameDT=off  OutDataTypeStr=boolean
  MATLAB Function : MATLAB Function  TreatAsAtomicUnit=on
  Relational Operator{,1..3,5..8} (8 alike) : RelationalOperator  Operator===  OutDataTypeStr=boolean  RndMeth=Simplest
  Relational Operator4 : RelationalOperator  OutDataTypeStr=boolean  RndMeth=Simplest
  Switch : Switch  Criteria=u2 ~= 0
  Switch1 : Switch  Criteria=u2 ~= 0
  Switch2 : Switch  Criteria=u2 > Threshold
  Unit Delay{,1..3} (4 alike) : UnitDelay  SampleTime=-1  HasFrameUpgradeWarning=on
  VTPM_Chkfin_flg : Outport
  wires:
  S1ID/1 -> MATLAB Function/1(S1ID)
  S2ID/1 -> MATLAB Function/2(S2ID)
  S3ID/1 -> MATLAB Function/3(S3ID)
  S4ID/1 -> MATLAB Function/4(S4ID)
  S1L/1 -> MATLAB Function/5(S1L)
  S2L/1 -> MATLAB Function/6(S2L)
  S3L/1 -> MATLAB Function/7(S3L)
  S4L/1 -> MATLAB Function/8(S4L)
  [VTPM_LFID_raw] -> Relational Operator/1
  VINP_ChkLFID_raw/1 -> Relational Operator/2
  VINP_ChkRFID_raw/1 -> Relational Operator1/2
  [VTPM_RFID_raw] -> Relational Operator1/1
  VINP_ChkLRID_raw/1 -> Relational Operator2/2
  [VTPM_LRID_raw] -> Relational Operator2/1
  VINP_ChkRRID_rawn5/1 -> Relational Operator3/2
  [VTPM_RRID_raw] -> Relational Operator3/1
  Relational Operator/1 -> Logical Operator/1
  Relational Operator1/1 -> Logical Operator/2
  Relational Operator2/1 -> Logical Operator/3
  Relational Operator3/1 -> Logical Operator/4
  VINP_ChkStorge_flg/1 -> Switch/2
  Data Type Conversion/1 -> [VTPM_LFID_raw]  "VTPM_LFID_raw"
  Data Type Conversion1/1 -> [VTPM_RFID_raw]  "VTPM_RFID_raw"
  Data Type Conversion2/1 -> [VTPM_LRID_raw]  "VTPM_LRID_raw"
  Data Type Conversion3/1 -> [VTPM_RRID_raw]  "VTPM_RRID_raw"
  MATLAB Function/3(LRID) -> Data Type Conversion2/1
  MATLAB Function/4(RRID) -> Data Type Conversion3/1
  MATLAB Function/1(LFID) -> Data Type Conversion/1
  MATLAB Function/2(RFID) -> Data Type Conversion1/1
  VTPM_Locdonetimes_cnt/1 -> Relational Operator4/1
  Relational Operator4/1 -> Logical Operator1/5
  Constant/1 -> Relational Operator4/2
  [VTPM_LFID_raw] -> Chart/1(VTPM_LFID_raw)
  [VTPM_RFID_raw] -> Chart/2(VTPM_RFID_raw)
  [VTPM_LRID_raw] -> Chart/3(VTPM_LRID_raw)
  [VTPM_RRID_raw] -> Chart/4(VTPM_RRID_raw)
  Chart/1(VTPM_ChkLFID_raw) -> [VTPM_ChkLFID_raw]
  Chart/2(VTPM_ChkRFID_raw) -> [VTPM_ChkRFID_raw]
  Chart/3(VTPM_ChkLRID_raw) -> [VTPM_ChkLRID_raw]
  Chart/4(VTPM_ChkRRID_raw) -> [VTPM_ChkRRID_raw]
  VTPM_ALLFin_flg/1 -> [VTPM_ALLFin_flg]
  [VTPM_ALLFin_flg] -> MATLAB Function/9(VTPM_ALLFin_flg)
  Logical Operator/1 -> Switch/1
  Relational Operator6/1 -> Logical Operator1/2
  [VTPM_LFID_raw] -> Relational Operator5/1
  Relational Operator7/1 -> Logical Operator1/3
  [VTPM_RRID_raw] -> Relational Operator8/1
  Relational Operator5/1 -> Logical Operator1/1
  Relational Operator8/1 -> Logical Operator1/4
  [VTPM_LRID_raw] -> Relational Operator7/1
  [VTPM_RFID_raw] -> Relational Operator6/1
  Logical Operator1/1 -> Switch/3
  Switch/1 -> Switch1/1, Logical Operator2/1
  Logical Operator2/1 -> [VTPM_SaveToRAM_flg]
  [VTPM_SaveToRAM_flg] -> Chart/5(VTPM_SaveToRAM_flg)
  [VTPM_ChkLFID_raw] -> Unit Delay1/1
  Unit Delay1/1 -> Relational Operator5/2
  [VTPM_ChkRFID_raw] -> Unit Delay/1
  Unit Delay/1 -> Relational Operator6/2
  [VTPM_ChkLRID_raw] -> Unit Delay2/1
  Unit Delay2/1 -> Relational Operator7/2
  [VTPM_ChkRRID_raw] -> Unit Delay3/1
  Unit Delay3/1 -> Relational Operator8/2
  [VTPM_ALLFin_flg] -> Switch1/2
  Constant1/1 -> Switch1/3
  Data Type Conversion4/1 -> VTPM_Chkfin_flg/1
  Switch1/1 -> Logical Operator3/1
  VINP_TPMSStorge_flg/1 -> Logical Operator3/2
  Switch2/1 -> Data Type Conversion4/1
  Logical Operator3/1 -> Switch2/3
  VINP_TPMSResButt_flg/1 -> Switch2/2
  Constant2/1 -> Switch2/1

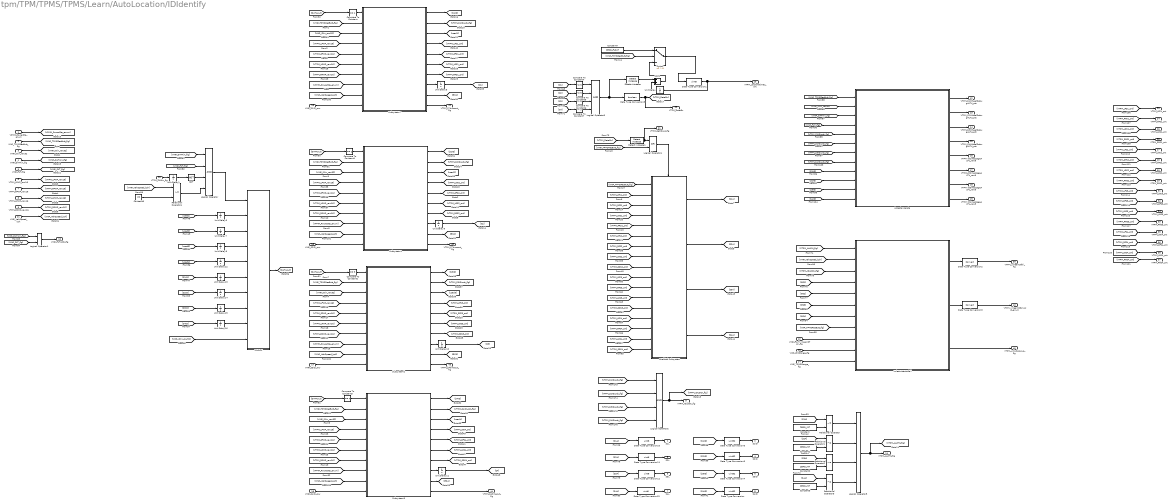
== system tpm/TPM/TPMS/TPMS/Learn/AutoLocation/IDIdentify ==
  VPMM_PowerSta_enum : Inport
  VINP_TPMSResButt_flg : Inport  Port=2
  VINP_IDin_raw32 : Inport  Port=3
  VINP_DATAin_flg : Inport  Port=4
  VINP_FAT_flg : Inport  Port=5
  VTPM_LFWP_raw16 : Inport  Port=6
  VTPM_RFWP_raw16 : Inport  Port=7
  VTPM_LRWP_raw16 : Inport  Port=8
  VTPM_RRWP_raw16 : Inport  Port=9
  VTPM_Chkfin_flg : Inport  Port=10
  VINP_VehSpeed_kph : Inport  Port=11
  VINP_FlashunlearnSfali_flg : Inport  Port=12
  VINP_ChkStorge_flg : Inport  Port=13
  VINP_TPMSStorge_flg : Inport  Port=14
  VINP_S1ID_raw : Inport  Port=15
  VINP_S2ID_raw : Inport  Port=16
  VINP_S3ID_raw : Inport  Port=17
  VINP_S4ID_raw : Inport  Port=18
  Acceptancerate : Subsystem
  Add1 : Sum
  Compare To Constant : simulink/Logic and Bit Operations/Compare To Constant  relop===  const=1  OutDataTypeStr=boolean
  Compare To Constant1 : simulink/Logic and Bit Operations/Compare To Constant  relop===  const=2  OutDataTypeStr=boolean
  Compare To Constant2 : simulink/Logic and Bit Operations/Compare To Constant  relop===  const=3  OutDataTypeStr=boolean
  Compare To Constant3 : simulink/Logic and Bit Operations/Compare To Constant  relop===  const=4  OutDataTypeStr=boolean
  Compare To Constant{4..7} (4 alike) : simulink/Logic and Bit Operations/Compare To Constant  relop=>=  const=9  OutDataTypeStr=boolean
  Constant{,1..3} (4 alike) : Constant  Value=ZERO_INT
  Constant4 : Constant  Value=ZERO_FLOAT
  Constant5 : Constant  Value=20  OutDataTypeStr=single
  Data Type Conversion{,4..6} (4 alike) : DataTypeConversion  OutDataTypeStr=uint32
  Data Type Conversion{1,10..13} (5 alike) : DataTypeConversion  OutDataTypeStr=uint8
  Data Type Conversion2 : DataTypeConversion
  Data Type Conversion3 : DataTypeConversion
  Data Type Conversion8 : DataTypeConversion  OutDataTypeStr=boolean
  Detect Increase : simulink/Logic and Bit Operations/Detect Increase  vinit=0.0  OutDataTypeStr=boolean
  Detect Increase1 : simulink/Logic and Bit Operations/Detect Increase  vinit=0.0  OutDataTypeStr=boolean
  Enabled Subsystem : Subsystem  TreatAsAtomicUnit=on
  IDLOCK : Stateflow chart  TreatAsAtomicUnit=on
  Logical Operator{,2..3,5} (4 alike) : Logic  Inputs=4  AllPortsSameDT=off  OutDataTypeStr=boolean
  Logical Operator1 : Logic  AllPortsSameDT=off  OutDataTypeStr=boolean
  Logical Operator4 : Logic  Operator=OR  AllPortsSameDT=off  OutDataTypeStr=boolean
  NOT : Logic  Operator=NOT  IconShape=distinctive  AllPortsSameDT=off  OutDataTypeStr=boolean
  Relational Operator{,1..3} (4 alike) : RelationalOperator  Operator=~=  OutDataTypeStr=boolean  RndMeth=Simplest
  Relational Operator4 : RelationalOperator  OutDataTypeStr=boolean  RndMeth=Simplest
  Subsystem1 : Subsystem
  Subsystem2 : Subsystem
  Subsystem3 : Subsystem
  Subsystem7 : Subsystem
  Switch : Switch  Criteria=u2 > Threshold
  Unit Delay{,1,5..16} (14 alike) : UnitDelay  SampleTime=-1  HasFrameUpgradeWarning=on
  "unlearnsensorfail " : Subsystem
  S1L : Outport
  S1ID : Outport  Port=2
  S2L : Outport  Port=3
  S2ID : Outport  Port=4
  S3L : Outport  Port=5
  S3ID : Outport  Port=6
  S4L : Outport  Port=7
  S4ID : Outport  Port=8
  VTPM_IDLOCK_flg : Outport  Port=9
  VINP_FATAND_flg : Outport  Port=10
  VTPM_ALLFIN_flg : Outport  Port=11
  VTPM_S1WheelDebugALTU_pct : Outport  Port=12
  VTPM_S2WheelDebugALTU_pct : Outport  Port=13
  VTPM_S3WheelDebugALTU_pct : Outport  Port=14
  VTPM_S4WheelDebugALTU_pct : Outport  Port=15
  VTPM_ID1messageALTU_raw8 : Outport  Port=16
  VTPM_ID2messageALTU_raw8 : Outport  Port=17
  VTPM_ID3messageALTU_raw8 : Outport  Port=18
  VTPM_ID4messageALTU_raw8 : Outport  Port=19
  VTPM_Locdonetimes_cnt : Outport  Port=20
  VTPM_SetIDLoc_flg : Outport  Port=21
  VTPM_DataEn : Outport  Port=22
  VTPM_LFS1_cnt : Outport  Port=23
  VTPM_RFS1_cnt : Outport  Port=24
  VTPM_RRS1_cnt : Outport  Port=25
  VTPM_LRS1_cnt : Outport  Port=26
  VTPM_LFS2_cnt : Outport  Port=27
  VTPM_RFS2_cnt : Outport  Port=28
  VTPM_RRS2_cnt : Outport  Port=29
  VTPM_LRS2_cnt : Outport  Port=30
  VTPM_LFS3_cnt : Outport  Port=31
  VTPM_RFS3_cnt : Outport  Port=32
  VTPM_RRS3_cnt : Outport  Port=33
  VTPM_LRS3_cnt : Outport  Port=34
  VTPM_LFS4_cnt : Outport  Port=35
  VTPM_RFS4_cnt : Outport  Port=36
  VTPM_RRS4_cnt : Outport  Port=37
  VTPM_LRS4_cnt : Outport  Port=38
  VTPM_unlearnSfali_flg : Outport  Port=39
  VTPM_unlearnSfailvalid_enum : Outport  Port=40
  VTPM_S1timeout_flg : Outport  Port=41
  VTPM_S2timeout_flg : Outport  Port=42
  VTPM_S3timeout_flg : Outport  Port=43
  VTPM_S4timeout_flg : Outport  Port=44
  VTPM_unlockpopup_flg : Outport  Port=45
  wires:
  VINP_TPMSResButt_flg/1 -> [VINP_TPMSResButt_flg]
  VTPM_RFWP_raw16/1 -> [VTPM_RFWP_raw16]
  NOT/1 -> Logical Operator/3
  VINP_IDin_raw32/1 -> [VINP_IDin_raw32]
  VTPM_RRWP_raw16/1 -> [VTPM_RRWP_raw16]
  VTPM_LRWP_raw16/1 -> [VTPM_LRWP_raw16]
  VTPM_LFWP_raw16/1 -> [VTPM_LFWP_raw16]
  Logical Operator2/1 -> [VTPM_IDLOCK_flg], VTPM_IDLOCK_flg/1
  [VTPM_S1IDLock_flg] -> Logical Operator2/1
  [VTPM_S2IDLock_flg] -> Logical Operator2/2
  [VTPM_S3IDLock_flg] -> Logical Operator2/3
  [VTPM_S4IDLock_flg] -> Logical Operator2/4
  Data Type Conversion/1 -> S4ID/1
  Data Type Conversion4/1 -> S3ID/1
  Data Type Conversion5/1 -> S2ID/1
  Data Type Conversion6/1 -> S1ID/1
  [S3ID] -> Unit Delay15/1
  [S4ID] -> Unit Delay16/1
  [used3] -> Unit Delay8/1
  [S2ID] -> Unit Delay14/1
  Unit Delay7/1 -> IDLOCK/3(used2)
  Unit Delay15/1 -> IDLOCK/8(IDout3)
  [VINP_IDin_raw32] -> IDLOCK/10(VINP_IDin_raw32)
  Unit Delay8/1 -> IDLOCK/4(used3)
  IDLOCK/1(DATAout) -> [DATAout]
  [used4] -> Unit Delay12/1
  [used1] -> Unit Delay6/1
  Unit Delay16/1 -> IDLOCK/9(IDout4)
  [used2] -> Unit Delay7/1
  [S1ID] -> Unit Delay13/1
  Unit Delay12/1 -> IDLOCK/5(used4)
  Unit Delay14/1 -> IDLOCK/7(IDout2)
  Unit Delay6/1 -> IDLOCK/2(used1)
  Unit Delay13/1 -> IDLOCK/6(IDout1)
  [VTPM_LFS2_cnt] -> Enabled Subsystem/6(VTPM_LFS2_cnt)
  [VTPM_RRS1_cnt] -> Enabled Subsystem/5(VTPM_RRS1_cnt)
  [VTPM_LRS3_cnt] -> Enabled Subsystem/12(VTPM_LRS3_cnt)
  [VTPM_RFS3_cnt] -> Enabled Subsystem/11(VTPM_RFS3_cnt)
  [VTPM_LRS2_cnt] -> Enabled Subsystem/8(VTPM_LRS2_cnt)
  [VTPM_LRS1_cnt] -> Enabled Subsystem/4(VTPM_LRS1_cnt)
  [VINP_TPMSResButt_flg] -> Enabled Subsystem/1(VINP_TPMSResButt_flg)
  [VTPM_RRS4_cnt] -> Enabled Subsystem/17(VTPM_RRS4_cnt)
  [VTPM_RFS1_cnt] -> Enabled Subsystem/3(VTPM_RFS1_cnt)
  [VTPM_LFS1_cnt] -> Enabled Subsystem/2(VTPM_LFS1_cnt)
  [VTPM_LFS3_cnt] -> Enabled Subsystem/10(VTPM_LFS3_cnt)
  [VTPM_RRS2_cnt] -> Enabled Subsystem/9(VTPM_RRS2_cnt)
  [VTPM_RRS3_cnt] -> Enabled Subsystem/13(VTPM_RRS3_cnt)
  [VTPM_LRS4_cnt] -> Enabled Subsystem/16(VTPM_LRS4_cnt)
  [VTPM_RFS2_cnt] -> Enabled Subsystem/7(VTPM_RFS2_cnt)
  [VTPM_LFS4_cnt] -> Enabled Subsystem/14(VTPM_LFS4_cnt)
  [VTPM_RFS4_cnt] -> Enabled Subsystem/15(VTPM_RFS4_cnt)
  Logical Operator/1 -> IDLOCK/1(VINP_DATAin_flg)
  Compare To Constant6/1 -> Logical Operator3/3
  Compare To Constant4/1 -> Logical Operator3/1
  Compare To Constant5/1 -> Logical Operator3/2
  Compare To Constant7/1 -> Logical Operator3/4
  [C1] -> Compare To Constant4/1
  [C2] -> Compare To Constant5/1
  [C3] -> Compare To Constant6/1
  [C4] -> Compare To Constant7/1
  Enabled Subsystem/1(S1L) -> [S1A]
  Enabled Subsystem/2(S2L) -> [S2A]
  Enabled Subsystem/3(S3L) -> [S3A]
  Enabled Subsystem/4(S4L) -> [S4A]
  Data Type Conversion13/1 -> S4L/1
  Logical Operator3/1 -> Detect Increase/1, Data Type Conversion8/1
  VINP_FAT_flg/1 -> [VINP_FAT_flg]
  VINP_DATAin_flg/1 -> [VINP_DATAin_flg]
  [VINP_FAT_flg] -> Logical Operator/2
  [VINP_DATAin_flg] -> Logical Operator/1
  [VINP_DATAin_flg] -> Logical Operator1/1
  [VINP_FAT_flg] -> Logical Operator1/2
  Logical Operator1/1 -> VINP_FATAND_flg/1
  Acceptancerate/1(S1WheelDebug_ALTU) -> VTPM_S1WheelDebugALTU_pct/1
  Acceptancerate/2(S2WheelDebug_ALTU) -> VTPM_S2WheelDebugALTU_pct/1
  Acceptancerate/3(S3WheelDebug_ALTU) -> VTPM_S3WheelDebugALTU_pct/1
  Acceptancerate/4(S4WheelDebug_ALTU) -> VTPM_S4WheelDebugALTU_pct/1
  Acceptancerate/5(ID1_message_ALTU) -> VTPM_ID1messageALTU_raw8/1
  Acceptancerate/6(ID2_message_ALTU) -> VTPM_ID2messageALTU_raw8/1
  Acceptancerate/7(ID3_message_ALTU) -> VTPM_ID3messageALTU_raw8/1
  Acceptancerate/8(ID4_message_ALTU) -> VTPM_ID4messageALTU_raw8/1
  [VINP_TPMSResButt_flg] -> Acceptancerate/1(VINP_TPMSResButt_flg)
  [VINP_IDin_raw32] -> Acceptancerate/2(VINP_IDin_raw32)
  [VINP_DATAin_flg] -> Acceptancerate/3(VINP_DATAin_flg)
  [VTPM_S1IDLock_flg] -> Acceptancerate/5(S1IDLock)
  [VINP_FAT_flg] -> Acceptancerate/4(VINP_FAT_flg)
  [S1ID] -> Acceptancerate/9(S1ID)
  [S2ID] -> Acceptancerate/10(S2ID)
  [VTPM_S2IDLock_flg] -> Acceptancerate/6(S2IDLock)
  [VTPM_S3IDLock_flg] -> Acceptancerate/7(S3IDLock)
  [VTPM_S4IDLock_flg] -> Acceptancerate/8(S4IDLock)
  [S3ID] -> Acceptancerate/11(S3ID)
  [S4ID] -> Acceptancerate/12(S4ID)
  [S1A] -> Data Type Conversion10/1
  Data Type Conversion10/1 -> S1L/1
  [S2A] -> Data Type Conversion11/1
  Data Type Conversion11/1 -> S2L/1
  [S3A] -> Data Type Conversion12/1
  Data Type Conversion12/1 -> S3L/1
  [S4A] -> Data Type Conversion13/1
  [S1ID] -> Data Type Conversion6/1
  [S2ID] -> Data Type Conversion5/1
  [S3ID] -> Data Type Conversion4/1
  [S4ID] -> Data Type Conversion/1
  VPMM_PowerSta_enum/1 -> [VPMM_PowerSta_enum]
  Detect Increase/1 -> Add1/1
  Unit Delay/1 -> Add1/2
  Unit Delay1/1 -> NOT/1
  VTPM_Chkfin_flg/1 -> Unit Delay1/1
  [VINP_TPMSResButt_flg] -> Logical Operator4/2
  [VTPM_DataEn] -> Detect Increase1/1
  Detect Increase1/1 -> VTPM_SetIDLoc_flg/1, Logical Operator4/1
  Logical Operator4/1 -> Enabled Subsystem/Enable
  [S1A] -> Relational Operator/1
  Constant/1 -> Relational Operator/2
  [S2A] -> Relational Operator1/1
  Constant1/1 -> Relational Operator1/2
  [S3A] -> Relational Operator2/1
  Constant2/1 -> Relational Operator2/2
  [S4A] -> Relational Operator3/1
  Constant3/1 -> Relational Operator3/2
  Relational Operator/1 -> Logical Operator5/1
  Relational Operator1/1 -> Logical Operator5/2
  Relational Operator2/1 -> Logical Operator5/3
  Relational Operator3/1 -> Logical Operator5/4
  Logical Operator5/1 -> [VTPM_ALLFIN_flg], VTPM_ALLFIN_flg/1
  Data Type Conversion8/1 -> VTPM_DataEn/1, [VTPM_DataEn]
  Constant4/1 -> Switch/1
  Data Type Conversion1/1 -> Unit Delay/1, VTPM_Locdonetimes_cnt/1  "VTPM_Locdonetimes_cnt"
  Switch/1 -> Data Type Conversion1/1
  Add1/1 -> Switch/3
  [VINP_TPMSResButt_flg] -> Switch/2
  Subsystem7/5(VTPM_RFS1_cnt) -> [VTPM_RFS1_cnt]
  [VTPM_LFWP_raw16] -> Subsystem7/4(VTPM_LFWP_raw16)
  [VTPM_LRWP_raw16] -> Subsystem7/6(VTPM_LRWP_raw16)
  [VTPM_RRWP_raw16] -> Subsystem7/7(VTPM_RRWP_raw16)
  [VPMM_PowerSta_enum] -> Subsystem7/8(VPMM_PowerSta_enum)
  Subsystem7/2(VTPM_S1IDLock_flg) -> [VTPM_S1IDLock_flg]
  [VINP_IDin_raw32] -> Subsystem7/3(VINP_IDin_raw32)
  [DATAout] -> Compare To Constant/1
  Subsystem7/1(IDOut) -> [S1ID]
  Subsystem7/3(Used) -> [used1]
  Subsystem7/6(VTPM_LRS1_cnt) -> [VTPM_LRS1_cnt]
  Subsystem7/8(C) -> Unit Delay5/1
  Subsystem7/7(VTPM_RRS1_cnt) -> [VTPM_RRS1_cnt]
  Unit Delay5/1 -> [C1]  "VTPM_C1_cnt"
  Compare To Constant/1 -> Subsystem7/1(VINP_DATAin_flg)
  [VTPM_RFWP_raw16] -> Subsystem7/5(VTPM_RFWP_raw16)
  Subsystem7/9(GS1) -> [GS1]
  Subsystem7/4(VTPM_LFS1_cnt) -> [VTPM_LFS1_cnt]
  [VINP_TPMSResButt_flg] -> Subsystem7/2(VINP_TPMSResButt_flg)
  Subsystem1/8(C) -> Unit Delay9/1
  Subsystem1/6(VTPM_LRS2_cnt) -> [VTPM_LRS2_cnt]
  Subsystem1/4(VTPM_LFS2_cnt) -> [VTPM_LFS2_cnt]
  Subsystem1/3(Used) -> [used2]
  Subsystem1/2(VTPM_S2IDLock_flg) -> [VTPM_S2IDLock_flg]
  Subsystem1/5(VTPM_RFS2_cnt) -> [VTPM_RFS2_cnt]
  [VTPM_LRWP_raw16] -> Subsystem1/6(VTPM_LRWP_raw16)
  [VTPM_RFWP_raw16] -> Subsystem1/5(VTPM_RFWP_raw16)
  Compare To Constant1/1 -> Subsystem1/1(VINP_DATAin_flg)
  [VTPM_RRWP_raw16] -> Subsystem1/7(VTPM_RRWP_raw16)
  [VINP_TPMSResButt_flg] -> Subsystem1/2(VINP_TPMSResButt_flg)
  [VTPM_LFWP_raw16] -> Subsystem1/4(VTPM_LFWP_raw16)
  [VINP_IDin_raw32] -> Subsystem1/3(VINP_IDin_raw32)
  Subsystem1/1(IDOut) -> [S2ID]
  Subsystem1/7(VTPM_RRS2_cnt) -> [VTPM_RRS2_cnt]
  [VPMM_PowerSta_enum] -> Subsystem1/8(VPMM_PowerSta_enum)
  Unit Delay9/1 -> [C2]  "VTPM_C2_cnt"
  [DATAout] -> Compare To Constant1/1
  Subsystem1/9(GS2) -> [GS2]
  Subsystem2/3(Used) -> [used3]
  [VINP_IDin_raw32] -> Subsystem2/3(VINP_IDin_raw32)
  Subsystem3/3(Used) -> [used4]
  [VPMM_PowerSta_enum] -> Subsystem2/8(VPMM_PowerSta_enum)
  [VINP_TPMSResButt_flg] -> Subsystem2/2(VINP_TPMSResButt_flg)
  [VTPM_RFWP_raw16] -> Subsystem2/5(VTPM_RFWP_raw16)
  Compare To Constant2/1 -> Subsystem2/1(VINP_DATAin_flg)
  [DATAout] -> Compare To Constant2/1
  [VTPM_LRWP_raw16] -> Subsystem2/6(VTPM_LRWP_raw16)
  Subsystem3/7(VTPM_RRS4_cnt) -> [VTPM_RRS4_cnt]
  Subsystem3/6(VTPM_LRS4_cnt) -> [VTPM_LRS4_cnt]
  Subsystem2/2(VTPM_S3IDLock_flg) -> [VTPM_S3IDLock_flg]
  Subsystem2/6(VTPM_LRS3_cnt) -> [VTPM_LRS3_cnt]
  [VTPM_LFWP_raw16] -> Subsystem3/4(VTPM_LFWP_raw16)
  Subsystem2/4(VTPM_LFS3_cnt) -> [VTPM_LFS3_cnt]
  [DATAout] -> Compare To Constant3/1
  Compare To Constant3/1 -> Subsystem3/1(VINP_DATAin_flg)
  Subsystem2/7(VTPM_RRS3_cnt) -> [VTPM_RRS3_cnt]
  [VTPM_LFWP_raw16] -> Subsystem2/4(VTPM_LFWP_raw16)
  Subsystem3/2(VTPM_S4IDLock_flg) -> [VTPM_S4IDLock_flg]
  [VINP_IDin_raw32] -> Subsystem3/3(VINP_IDin_raw32)
  Subsystem3/4(VTPM_LFS4_cnt) -> [VTPM_LFS4_cnt]
  Subsystem2/8(C) -> Unit Delay10/1
  Subsystem3/8(C) -> Unit Delay11/1
  [VPMM_PowerSta_enum] -> Subsystem3/8(VPMM_PowerSta_enum)
  Unit Delay11/1 -> [C4]  "VTPM_C4_cnt"
  [VTPM_LRWP_raw16] -> Subsystem3/6(VTPM_LRWP_raw16)
  [VINP_TPMSResButt_flg] -> Subsystem3/2(VINP_TPMSResButt_flg)
  Subsystem2/5(VTPM_RFS3_cnt) -> [VTPM_RFS3_cnt]
  Subsystem2/9(GS3) -> [GS3]
  [VTPM_RFWP_raw16] -> Subsystem3/5(VTPM_RFWP_raw16)
  Subsystem3/9(GS4) -> [GS4]
  Subsystem2/1(IDOut) -> [S3ID]
  [VTPM_RRWP_raw16] -> Subsystem3/7(VTPM_RRWP_raw16)
  [VTPM_RRWP_raw16] -> Subsystem2/7(VTPM_RRWP_raw16)
  Unit Delay10/1 -> [C3]  "VTPM_C3_cnt"
  Subsystem3/5(VTPM_RFS4_cnt) -> [VTPM_RFS4_cnt]
  Subsystem3/1(IDOut) -> [S4ID]
  [VTPM_IDLOCK_flg] -> "unlearnsensorfail "/3(VTPM_IDLOCK_flg)
  [GS1] -> "unlearnsensorfail "/4(GS1)
  [GS4] -> "unlearnsensorfail "/7(GS4)
  [GS3] -> "unlearnsensorfail "/6(GS3)
  [VTPM_ALLFIN_flg] -> "unlearnsensorfail "/1(VTPM_ALLFIN_flg)
  [GS2] -> "unlearnsensorfail "/5(GS2)
  [VINP_TPMSResButt_flg] -> "unlearnsensorfail "/8(VINP_TPMSResButt_flg)
  "unlearnsensorfail "/1(VTPM_unlearnSfali_flg) -> Data Type Conversion2/1
  Data Type Conversion2/1 -> VTPM_unlearnSfali_flg/1
  VINP_FlashunlearnSfali_flg/1 -> "unlearnsensorfail "/9(VINP_FlashunlearnSfali_flg)
  VINP_ChkStorge_flg/1 -> "unlearnsensorfail "/10(VINP_ChkStorge_flg)
  VINP_TPMSStorge_flg/1 -> "unlearnsensorfail "/11(VINP_TPMSStorge_flg)
  Data Type Conversion3/1 -> VTPM_unlearnSfailvalid_enum/1
  "unlearnsensorfail "/2(VTPM_unlearnSfailvalid_enum) -> Data Type Conversion3/1
  Constant5/1 -> Relational Operator4/2
  Relational Operator4/1 -> Logical Operator/4
  [VINP_VehSpeed_kph] -> Relational Operator4/1
  VINP_VehSpeed_kph/1 -> [VINP_VehSpeed_kph]
  [VINP_VehSpeed_kph] -> "unlearnsensorfail "/2(VINP_VehSpeed_kph)
  [VINP_VehSpeed_kph] -> Subsystem7/9(VINP_VehSpeed_kph)
  [VINP_VehSpeed_kph] -> Subsystem1/9(VINP_VehSpeed_kph)
  [VINP_VehSpeed_kph] -> Subsystem2/9(VINP_VehSpeed_kph)
  [VINP_VehSpeed_kph] -> Subsystem3/9(VINP_VehSpeed_kph)
  VINP_S1ID_raw/1 -> Subsystem7/10(VINP_S1ID_raw)
  VINP_S2ID_raw/1 -> Subsystem1/10(VINP_S2ID_raw)
  VINP_S3ID_raw/1 -> Subsystem2/10(VINP_S3ID_raw)
  VINP_S4ID_raw/1 -> Subsystem3/10(VINP_S4ID_raw)
  Subsystem7/10(VTPM_S1timeout_flg) -> VTPM_S1timeout_flg/1
  Subsystem1/10(VTPM_S2timeout_flg) -> VTPM_S2timeout_flg/1
  Subsystem2/10(VTPM_S3timeout_flg) -> VTPM_S3timeout_flg/1
  Subsystem3/10(VTPM_S4timeout_flg) -> VTPM_S4timeout_flg/1
  [VTPM_RFS1_cnt] -> VTPM_RFS1_cnt/1
  [VTPM_LFS1_cnt] -> VTPM_LFS1_cnt/1
  [VTPM_LRS1_cnt] -> VTPM_LRS1_cnt/1
  [VTPM_RRS1_cnt] -> VTPM_RRS1_cnt/1
  [VTPM_LFS2_cnt] -> VTPM_LFS2_cnt/1
  [VTPM_RFS2_cnt] -> VTPM_RFS2_cnt/1
  [VTPM_LRS2_cnt] -> VTPM_LRS2_cnt/1
  [VTPM_RRS2_cnt] -> VTPM_RRS2_cnt/1
  [VTPM_LFS3_cnt] -> VTPM_LFS3_cnt/1
  [VTPM_RFS3_cnt] -> VTPM_RFS3_cnt/1
  [VTPM_LRS3_cnt] -> VTPM_LRS3_cnt/1
  [VTPM_RRS3_cnt] -> VTPM_RRS3_cnt/1
  [VTPM_RRS4_cnt] -> VTPM_RRS4_cnt/1
  [VTPM_LRS4_cnt] -> VTPM_LRS4_cnt/1
  [VTPM_RFS4_cnt] -> VTPM_RFS4_cnt/1
  [VTPM_LFS4_cnt] -> VTPM_LFS4_cnt/1
  "unlearnsensorfail "/3(VTPM_unlockpopup_flg) -> VTPM_unlockpopup_flg/1
